simulink model "System_Modell"  (R2018a)
settings: Solver=FixedStepAuto  StartTime=0.0  StopTime=inf  FixedStep=1/f  RelTol=1e-3
values from neighbouring files (symbols this model uses):
  f = 10000    [System_Init.m]
(part 4 of 8)

== matlab function System_Modell/Motor_1/Schnittstelle_0/Recv_2 ==
  data: status input double size=1; clock input double size=1; lenS_1 input; lenS_2 input; lenR input; Rx_2_signal input boolean size=1; Rx_2_data input double size=[1 100]; recv_signal_2 output boolean; recv_package_2 output double size=[1 98]; Send_Buffer_1 data_store_memory; Send_Buffer_2 data_store_memory; T_send_1 data_store_memory; T_recv_1 data_store_memory; De_1 data_store_memory; De_sum_1 data_store_memory; Address data_store_memory; Recv_Buffer data_store_memory; Address_2 data_store_memory; Address_1 data_store_memory; De_sum_2 data_store_memory; Handshake_1 data_store_memory; De_2 data_store_memory; Handshake_2 data_store_memory; T_recv_2 data_store_memory; T_send_2 data_store_memory
% Name: Rx_2

% -------------------------------------------------------------------------------------
% Funktionalitäten:
% Im Init-Prozess
%   1. Handshake durch zu führen
%       103...Handshake ask --> 104 in Send_Buffer_1 additieren
%       104...Handshake answer --> Handshake success
%   2. Delay-Zeit berechnen
%       105...Delay begin --> 106 in Send_Buffer_1 additieren
%       106...Delay end --> Delay_Zeit berechnen
%   3. Sum-Delay-Zeit berechnen
%       107, Receiver = meine Addresse --> Sum_Delay_Zeit berechnen
%       107, Receiver ~= meine Addresse --> Daten in Send_Buffer_2 additieren
% Im normalen Prozess
%   4. Receiver = meine Addresse --> in Recv_Buffer additieren
%   5. Receiver = 255 --> Broadcast --> in Recv_Buffer && Send_Buffer_2 additieren
%   6. Receiver ~= meine Addresse --> in Send_Buffer_2 additieren

% -------------------------------------------------------------------------------------
% Input && Output
% status - status of 'Schnittstelle'
% clock - simulation time
% lenS_2/len_1/lenR - meaningful length of Send_Buffer_2/Send_Buffer_1/Recv_Buffer
% Rx_2_data - from Rx_2 received data
% recv_package_2 - data to send to chart or store in Send_Buffer_2
    % in Init-process, recv_package_2 need to be sent to chart
    % in normal-process, recv_package_2 need to garther all 'to be transmmited' datablock, and store in Send_Buffer_2

function [recv_signal_2, recv_package_2] = Rx_2(status, clock,lenS_1, lenS_2, lenR, Rx_2_signal, Rx_2_data)

global Send_Buffer_2
global Send_Buffer_1
global T_send_2
global T_recv_2
global De_2
%global De_1
global De_sum_2
global Address
global Address_2
%global Address_1
global Recv_Buffer
global Handshake_2

recv_signal_2 = false;
recv_package_2 = zeros(1,98);       % one datablock = [1x7]

lenr = 1;                           % path to write data into recv_package_2

if Rx_2_signal
    a = find(Rx_2_data==102,1);
    len = a(1);
    if ~isempty(len)
        mod_ = mod(len-2,7);
        len_ = ceil((len - 2) / 7);                                 % Round toward positive infinity
    end
    
	if ((mod_ == 0) && (len_ >= 1))                             % package contains at least one datablock
        switch status
            case 1                                              % Handshake
                for i=1:len_
                    switch Rx_2_data(7*i-3)                          % Da.cmd
                        case 103                                % Handshake ask --> send answer
                            check = check_X(104, Address, Send_Buffer_1);
                            if ((Rx_2_data(7*i-5) ~= 0) && (Rx_2_data(7*i-4) == 0) && ~Handshake_2 && ~check)
                                Address_2 = Rx_2_data(7*i-5);
                                Send_Buffer_1(lenS_1:lenS_1+7) = [Address, Address_2, 104, zeros(1,4), 102];
                            end
                        case 104                                % Handshake answer --> Handshake success --> no more send
                            if ((Rx_2_data(7*i-5) ~= 0) && (Rx_2_data(7*i-4) == Address) && ~Handshake_2)
                                Address_2 = Rx_2_data(7*i-5);        % Address of the Host in the Direction_2
                                recv_package_2(lenr:lenr+6) = Rx_2_data(7*i-5:7*i+1);    % [_,_,104,_,_,_,_] = [1x7]
                                lenr = lenr + 7;
                                recv_signal_2 = true;
                            end
                    end
                end

            case 2                                              % Delay_Time_Caculation
                for j=1:len_
                    switch Rx_2_data(7*j-3)                          % Da.cmd
                        case 103                                % Handshake ask --> send answer
                            check = check_X(104, Address, Send_Buffer_1);
                            if ((Rx_2_data(7*j-5) ~= 0) && (Rx_2_data(7*j-4) == 0) && ~Handshake_2 && ~check)
                                Address_2 = Rx_2_data(7*j-5);
                                Send_Buffer_1(lenS_1:lenS_1+7) = [Address, Address_2, 104, zeros(1,4), 102];
                            end
                        case 105                                % Delay ask --> send answer
                            check = check_X(106, Address, Send_Buffer_1);
                            if (isequal(Rx_2_data(7*j-5:7*j-4),[Address_2, Address]) && Handshake_2 && ~check) % check Sender & Receiver
                                Send_Buffer_1(lenS_1:lenS_1+7) = [Address, Address_2, 106, zeros(1,4), 102];
                            end
                        case 106                                % Delay answer --> caculate the time --> no more send
                            if ((isequal(Rx_2_data(7*j-5:7*j-3),[Address_2, Address, 106])) && (De_2 <= 0) && (T_send_2 > 0))
                                T_recv_2 = clock;
                                De_2 = T_recv_2 - T_send_2;
                                T_send_2 = 0;
                                T_recv_2 = 0;
                            end
                    end
                end

            case 3                                              % Sum_Delay_Caculation
                for h=1:len_
                    switch Rx_2_data(7*h-3)
                        case 103                                % Handshake ask --> send answer
                            check = check_X(104, Address, Send_Buffer_1);
                            if ((Rx_2_data(7*h-5) ~= 0) && (Rx_2_data(7*h-4) == 0) && ~Handshake_2 && ~check)
                                Address_2 = Rx_2_data(7*h-5);
                                Send_Buffer_1(lenS_1:lenS_1+7) = [Address, Address_2, 104, zeros(1,4), 102];
                            end
                        case 105                                % Delay ask --> send answer
                            check = check_X(106, Address, Send_Buffer_1);
                            if (isequal(Rx_2_data(7*h-5:7*h-4),[Address_2, Address]) && Handshake_2 && ~check) % check Sender & Receiver
                                Send_Buffer_1(lenS_1:lenS_1+7) = [Address, Address_2, 106, zeros(1,4), 102];
                            end   
                        case 107
                            if (isequal(Rx_2_data(7*h-5:7*h-4),[Address, Address]) && (De_sum_2 <= De_2) && (T_send_2 > 0))                   % Sum_Delay --> caculate the time --> no more send
                                T_recv_2 = clock;
                                De_sum_2 = T_recv_2 - T_send_2;
                                T_send_2 = 0;
                                T_recv_2 = 0;
                            elseif ((isequal(Rx_2_data(7*h-5),Rx_2_data(7*h-4))) && (Rx_2_data(7*h-5) ~= Address))
                                check = check_Y(Rx_2_data(7*h-5:7*h), recv_package_2) || check_Y(Rx_2_data(7*h-5:7*h), Send_Buffer_2);
                                if ~check
                                    recv_package_2(lenr:lenr+6) = Rx_2_data(7*h-5:7*h+1)';
                                    lenr = lenr + 7;
                                end
                            end
                    end
                end
                Send_Buffer_2(lenS_2:lenS_2+lenr-1) = [recv_package_2(1:lenr-1),102];           % 前提：lenS更新速度比当前更新快

            case 4                                               % normal communication between all Hosts
                for k=1:len_
                    switch Rx_2_data(7*k-3)
                        case 103                                % Handshake ask --> send answer
                            check = check_X(104, Address, Send_Buffer_1);
                            if ((Rx_2_data(7*k-5) ~= 0) && (Rx_2_data(7*k-4) == 0) && ~Handshake_2 && ~check)
                                Address_2 = Rx_2_data(7*k-5);
                                Send_Buffer_1(lenS_1:lenS_1+7) = [Address, Address_2, 104, zeros(1,4), 102];
                            end
                        case 105                                % Delay ask --> send answer
                            check = check_X(106, Address, Send_Buffer_1);
                            if (isequal(Rx_2_data(7*k-5:7*k-4),[Address_2, Address]) && Handshake_2 && ~check) % check Sender & Receiver
                                Send_Buffer_1(lenS_1:lenS_1+7) = [Address, 0, 106, zeros(1,4), 102];
                            end
                        case 107
                            if ((isequal(Rx_2_data(7*k-5),Rx_2_data(7*k-4))) && (Rx_2_data(7*k-5) ~= Address))
                                check = check_Y(Rx_2_data(7*k-5:7*k), recv_package_2) || check_Y(Rx_2_data(7*k-5:7*k), Send_Buffer_2);
                                if ~check
                                    recv_package_2(lenr:lenr+6) = Rx_2_data(7*k-5:7*k+1)';
                                    lenr = lenr + 7;
                                end
                            end
                        otherwise
                            if ((Rx_2_data(7*k-5) ~= Address) && (Rx_2_data(7*k-4) == Address))   % Datablock sent to me --> store in Recv_Buffer
                                check = check_Y(Rx_2_data(7*k-5:7*k), Recv_Buffer');
                                if ~check
                                    Recv_Buffer(lenR+1,:) = Rx_2_data(7*k-5:7*k+1);
                                end
                            elseif ((Rx_2_data(7*k-5) ~=Address) && (Rx_2_data(7*k-4) == 255))    % Datablock is as a Broadcast --> store in Recv_Buffer && Send_Buffer_2
                                check = check_Y(Rx_2_data(7*k-5:7*k), Recv_Buffer');
                                if ~check
                                    Recv_Buffer(lenR+1,:) = Rx_2_data(7*k-5:7*k+1);
                                end
                                check = check_Y(Rx_2_data(7*k-5:7*k), recv_package_2) || check_Y(Rx_2_data(7*k-5:7*k), Send_Buffer_2);
                                if ~check
                                    recv_package_2(lenr:lenr+6) = Rx_2_data(7*k-5:7*k+1)';
                                    lenr = lenr + 7;
                                end
                            elseif ((Rx_2_data(7*k-4) ~= Address) && (Rx_2_data(7*k-4) ~= 255))   % Datablock not sent to me --> to transmmit --> store in Send_Buffer_2
                                check = check_Y(Rx_2_data(7*k-5:7*k), recv_package_2) || check_Y(Rx_2_data(7*k-5:7*k), Send_Buffer_2);
                                if ~check
                                    recv_package_2(lenr:lenr+6) = Rx_2_data(7*k-5:7*k+1)';
                                    lenr = lenr + 7;
                                end
                            end
                    end
                end
                Send_Buffer_2(lenS_2:lenS_2+lenr-1) = [recv_package_2(1:lenr-1),102];
        end
	elseif mod_ ~= 0
        fprintf("Eroor: Package length not avalueable!");
	end
end

end

% check_X: to check if Data contains a Datablock with CMD and adr
function y = check_X(CMD, adr, Data)          % y: boolean; x: double, [1x100];

x = find(Data==CMD);
y = (~isempty(x));

if y
    y = y && (Data(1,x(1)-2) == adr);
end

end

% check_Y: to check if Data contains data
function y = check_Y(data, Data)          % y: boolean; data: double, [1x6];

x = find(Data==data(3));
y = (~isempty(x));
if y
    for i=1:length(x)
        if(isequal(Data(x(i)-2:x(i)+3),data))
            y = true;
            break
        else
            y = false;
        end
    end
end

end

== matlab function System_Modell/Motor_1/Schnittstelle_0/Send_Telegram/Send_Telegram_1 ==
  data: status input double size=1; clock input double; lenS_1 input; impulse input boolean size=1; Tx_1_signal output boolean size=1; Tx_1_data output double size=[1,100]; send_1_old input boolean size=1; T_send_1 data_store_memory; T_send_2 data_store_memory; Send_Buffer_1 data_store_memory; Send_Buffer_2 data_store_memory; De_1 data_store_memory; De_2 data_store_memory; De_sum_1 data_store_memory; De_sum_2 data_store_memory; Address data_store_memory
% Name: send_telegram
% Funktionalität:
% Datenpacket in Send_Buffer_1 und Send_Buffer2 zyklisch transferieren.
% Die Zykluszeit lautet 10ms

function [Tx_1_signal, Tx_1_data] = send_telegram_1(status, clock, lenS_1, impulse, send_1_old)

global Send_Buffer_1
global De_1
global De_sum_1
global T_send_1
global Address

timer_1 = 0;

if send_1_old
    % The Send_Signal lasts for only one period. Then it need to be shut down.
    Tx_1_signal = false;
    Tx_1_data = [101,102,zeros(1,98)];
else
    % No Error + send-signal already shut down + Impulse-Signal --> OK! Let's send the telegram!
    h1 = ceil((lenS_1 - 2) / 7);
    if ((status > 0) && (~send_1_old) && impulse && (h1 > 0))
        % Before send, we need check if we need to do something else. For example: 'start the Timer' or 'caculate a new De in each datablock'
        switch status
            case 2                                              % Delay time caculation
                if ~isempty(find(Send_Buffer_1==105,1))                     % check if there is a 105-cmd in Send_Buffer,if so, timer need to be started
                    timer_1 = 1;
                end

            case 3                                              % Sum_Delay caculation
                for i1=1:h1
                    if isequal([Send_Buffer_1(7*i1-5:7*i1-3),De_sum_1],[Address,Address,107,0])     % check if there is a 107-cmd in Send_Buffer
                        timer_1 = 1;
                        break
                    end
                end

            case 4
                for i1=1:h1                                                    % recaculate the Delay time for each datablock
                    Send_Buffer_1(7*i1+1) = Send_Buffer_1(7*i1+1) + De_1;
                end
        end
        
        % Now we can send the telegram!!
        Tx_1_data = Send_Buffer_1;                                  % send data
        Tx_1_signal = true;
        
        % remember the send-time if necessary
        if timer_1 == 1
            T_send_1 = clock;
        end
        
        % clear the data in Send_Buffer after sending
        Send_Buffer_1 = [101,102,zeros(1,98)];

    else
        Tx_1_signal = false;
        Tx_1_data = [101,102,zeros(1,98)];
    end
end

end

== matlab function System_Modell/Motor_1/Schnittstelle_0/Send_to_Host ==
  data: signal output boolean size=1; package output double; Recv_Buffer data_store_memory; Filter data_store_memory; lenR input; lenF input; signal_old input
% Name: Send_to_Host
% Funktionalitäten:
% 1. Erste Zeile der Nachricht von Recv_Buffer in Filter prüfen
% 2. nicht wiederholte Nachricht an Host senden
% 3. wiederholte Nachricht in Filter löschen
% 4. gesendete Nachricht in Filter kopieren
% 5. folgende Nachrichten eine Zeile nach oben verschoben


function [signal, package] = send_to_Host(lenR, lenF, signal_old)

global Recv_Buffer          % Package-List, which will be sent to the Host
global Filter               % Package-List, which has been sent to the Host

package = zeros(1,7);
check = 0;

if signal_old               % signal can only last for one periode
    signal = false;
    package = zeros(1,7);

else                        % signal inactiv --> now we can send new data to host.
    if (lenR >= 1)
        if lenF >= 1        % check in Filter
            for i=1:lenF        % check if the same message sent before
                if isequal(Recv_Buffer(1,:),Filter(i,:))
                    check = i;
                    break
                else
                    check = 0;
                end
            end
        end
        
        if check ~= 0       % same message in Filter found --> delete the message in Recv_Buffer and Filter
            signal = false;
            package = zeros(1,7);
            Filter(check:lenF-1,:) = Filter(check+1:lenF,:);
            Filter(lenF,:) = zeros(1,7);
            Recv_Buffer(1:lenR-1,:) = Recv_Buffer(2:lenR,:);
            Recv_Buffer(lenR,:) = zeros(1,7);
        else                % same message in Filter not found --> send to Host --> copy the message in Filter delete it in Recv_Buffer
            package = Recv_Buffer(1,:);
            signal = true;
            Filter(lenF+1,:) = Recv_Buffer(1,:);    % copy
            Recv_Buffer(1:lenR-1,:) = Recv_Buffer(2:lenR,:);    % delete
            Recv_Buffer(lenR,:) = zeros(1,7);
        end
    else
        signal = false;
        package = zeros(1,7);
    end
end


end

== stateflow chart System_Modell/Motor_1/Schnittstelle_0/Status ==
  state Init_0
    entry:	status=0;
    Handshake_1=false;
    Handshake_2=false;
    De_1 = 0;
    De_2 = 0;
    De_sum_1 = 0;
    De_sum_2 = 0;
    Filter(1,:) = zeros(1,7);
  state Error
    entry: status=-2;
  note: 未初始化全局变量
  state Init_1_Handshake
    entry: status=1;
  state Init_2_Delay_Time
    entry:	status=2;
  state Init_3_Sum_Delay_Time
    entry:	status=3;
  state Run
    entry: status=4;
  (default) -> Init_0
  Error -> Init_0 : [~Error_Signal]
  Init_0 -> Init_1_Handshake
  Init_1_Handshake -> Error [order 3] : [Error_Signal]
  Init_1_Handshake -> (junction 75) [order 1] : [recv_signal_1]
  (junction 75) -> Init_1_Handshake : [recv_data_1(1,3)==104]{Handshake_1 = true;}
  Init_1_Handshake -> (junction 77) [order 2] : [recv_signal_2]
  (junction 77) -> Init_1_Handshake : [recv_data_2(1,3)==104]{Handshake_2 = true;}
  Init_1_Handshake -> Init_2_Delay_Time [order 4] : [Handshake_1 && Handshake_2 && Address_1 > 0 && Address_2 > 0]
  Init_2_Delay_Time -> Error [order 2] : [Error_Signal]
  Init_2_Delay_Time -> Init_3_Sum_Delay_Time [order 1] : [De_1>0 && De_2>0]
  Init_3_Sum_Delay_Time -> Error [order 2] : [Error_Signal]
  Init_3_Sum_Delay_Time -> Run [order 1] : [De_sum_1 > De_1 && De_sum_2 > De_2]
  Run -> Error : [Error_Signal]
  data: status output double size=1; Error_Signal input boolean size=1; recv_signal_1 input boolean size=1; recv_data_1 input double; Handshake_1 data_store_memory size=1; Handshake_2 data_store_memory size=1; De_1 data_store_memory; De_2 data_store_memory; De_sum_1 data_store_memory; De_sum_2 data_store_memory; recv_signal_2 input boolean; recv_data_2 input double; Address_1 data_store_memory; Address_2 data_store_memory; Filter data_store_memory

== stateflow chart System_Modell/Motor_2/CommSM_1/Status_Control ==
  state Init
    entry: 	status=1;
    send_AT_package=[Adresse, zeros(1,6)];
    send_signal=false;
    send_MotionSM=[0,0];
  state Aus
    entry: status=0;
  state Ein
    state State_Control [parallel]
      settings: executionOrder=1
      note: % Protokoll
          | % SummenTelegramm = [HDR, SDT, END]
          | %HDR: header, SDT: Summen-Daten-Telegramm, END: Ender
          |
          | % SDT = [SDT_7, SDT_1, SDT_2, SDT_3]
          | % SDT_i = [Da_i, De_i]
          | %Da: Data, De: Delay
          | %i...{1,2,3,7} %7...GSM, 1-3...CommSM1-3
          |
          | % Da_i = [sender, receiver, cmd, N, ZP, ZP_status]
          | %sender,receiver...{1,2,3,7,255} %255...Broadcast
          | %cmd: 1...addP, 2...getP, 3...setS, 4...getS
          | %ZP_status: 0...none, 1...wait, 2...active, 3...done, 4...error
          |
          | % Da_i = [sender, receiver, cmd, N, s , s _status]
          | %cmd: 5 ...negO
          | % s _status: 0...none, 1...negotiation, 2...excute, 3...done
      note: 问题
          | 如何检测下一个新的ZP
      state send_AT_2_GSM
        entry:	status=16;
        permission=true;
        send_AT_package=[Adresse, 7, 113, ZPT(N,1:3), 0];
        %AT=[CommSM, GSM, setS, n, ZP, done];
        send_signal=true;
      state Free
        entry:	status=2;
      state Arrival
        entry:	status=15;
        ZPT(N,3)=3;
      state check_ZPT
        entry:	status=3;
        ZPT(N,3)=2;	      % status='active'
      state wait_arrival
        entry: status=14
      state send_Status_activ
        entry:	status=4;
        permission = true;
        send_AT_package = [Adresse, 7, 113, ZPT(N,1:3), 0];
        % AT=[CommSM, GSM, setS, n, ZP, activ];
        send_signal = true;
      state check_ZP
        entry: 	status=5;
        s=checkZP(ZZP_old, Adresse, N);
        % s-range: [0, 100], ZZP_old: ZZP for last loop
      state MotionSM
        entry:	status=13;
        send_MotionSM=[3, ZZPT(Adresse,2)];	%excute ZZP
        a = ZPT(N,2); b = ZZPT(Adresse,2);
      state send_nego_1
        entry: 	status=6;
        permission = true;
        send_AT_package=[Adresse, 255, 115, ZPT(N,1), s, 1, 0];
        % AT=[CommSM, Broadcast, negO, n, s, nego];
        send_signal=true;
      state Nego_wait
        entry: 	status=7;
      state send_excu
        entry:	status=12;
        permission = true;
        send_AT_package = [Adresse, 255, 115, ZPT(N,1), ZZPT(Adresse, 4), 2, 0];
        %AT=[CommSM, Broadcast, negO, n, s, excu];
        send_signal = true;
      state Wait_excution
        entry:	status=11;
        send_MotionSM=[1, ZZPT(Adresse,2)]; %set ZZP
      state s_Compair
        entry: 	status=8;
        s_new=s_compair(Adresse);
      state status_excution
        entry: 	status=10;
        ZZPT(Adresse,4)=2; %excu
      state ZZP_new
        entry:	status=9;
        ZZPT(Adresse,3)=s_new;
        ZZPT(Adresse,2)=AP+(ZPT(N,2)-AP)*(s_new/100);
      (default) -> Free
      send_AT_2_GSM -> Free : [send_done]{send_signal=false; permission = false;}
      Free -> check_ZPT : % status ='wait' && MotionSM kein Fehler
          | [N>0 && ZPT(N,3)==1 && status_MotionSM>=1]{send_signal = false;}
      (junction 77) -> send_AT_2_GSM : [~permission]
      Arrival -> (junction 77)
      (junction 121) -> (junction 77)
      wait_arrival -> Arrival : % ZP == ZZP -> wait until ZP == AP
          | [isequal([ZPT(N,2), status_MotionSM],[AP, 2])]
          | {ZZPT=zeros(3,4);}
      check_ZPT -> send_Status_activ : [ZPT(N,3)==2 && ~permission]
      MotionSM -> wait_arrival [order 2] : % ZP == ZZP -> ZP will be arrived & no next ZP -> end
          | [status_MotionSM==3 && a==b && isempty(find(ZPT(:,3)==1,1))]
          | {send_MotionSM=zeros(1,2)}
      (junction 116) -> (junction 99)
      (junction 148) -> (junction 116)
      send_Status_activ -> (junction 99) : [send_done]{send_signal = false; permission = false;}
      (junction 99) -> check_ZP
      MotionSM -> (junction 116) [order 1] : % ZP~=ZZP -> ZP will not be arrived -> negotiate again
          | [status_MotionSM==3 && a~=b]
          | {ZZP_old = ZZPT(Adresse,2); ZZPT = zeros(3,4);}
      MotionSM -> (junction 148) [order 3] : [false]
          | % ZP = ZZP -> ZP will be arrived -> new ZP wait to negotiate -> loop
          | %[status_MotionSM==3 && a==b && ~isempty(find(ZPT(:,3)==1,1))]
          | %{ZZP_old = ZZPT(Adresse,2); ZZPT = zeros(3,4)}
      check_ZP -> send_nego_1 : [~permission]
      (junction 146) -> MotionSM : % Motor stoped
          | [status_MotionSM==2]
      (junction 216) -> (junction 146) : % all axis excuteable && received ZZP from MotionSM
          | [isequal(ZZPT(1:3,4),[2;2;2]) && isequal(data_from_MotionSM(1:2),[2,ZZPT(Adresse,2)])]
          | {ZZP_old=0;}
      send_nego_1 -> Nego_wait : [send_done]{s=0; send_signal=false; permission = false;}
      send_excu -> (junction 216) : [send_done]{send_signal=false; permission = false;}
      Nego_wait -> (junction 121) [order 1] : % ZP = AP, ZP schon erreicht
          | [ZPT(N,3)==3]
      Nego_wait -> (junction 134) [order 2] : % ZP~=AP, ZP "activ"
          | [ZPT(N,3)==2]
      Wait_excution -> send_excu : [~permission]
      (junction 134) -> s_Compair : % ob ZZPT komplett erfüllt
          | [isequal(ZZPT(1:3,1),[1,1,1]')]
      status_excution -> Wait_excution : [status_MotionSM>=2]  % 2 or 3
      s_Compair -> (junction 79)
      (junction 66) -> status_excution : {s_new=0;}
      (junction 79) -> (junction 66) [order 2] : [s_new>=ZZPT(Adresse,3)]
      (junction 79) -> ZZP_new [order 1] : [s_new<ZZPT(Adresse,3)]
      ZZP_new -> (junction 66)
    state Send [parallel]
      settings: executionOrder=2
      state wait
      state send
        entry: permission = true;
        send_AT_package = [Adresse, 7, 2, ZPT(n-1,1:3),0];
        send_signal = true;
      (default) -> wait
      wait -> (junction 181) : % Requirement to respond GSM
          | [respond]
      send -> wait : % send done
          | [send_done]{respond = false;send_signal = false; permission = false;}
      (junction 181) -> send : % permission to use send_port
          | [~permission]
  state Error
    entry: status=-1;
  (default) -> Aus
  Aus -> Init : [EinAus && ~NotAus && ~ErrorSignal]
  Init -> Aus [order 2] : [~EinAus]
  Init -> Error [order 3] : [NotAus]
  Error -> Aus [order 1] : [~EinAus]
  Ein -> Aus [order 1] : [~EinAus]
  Error -> Init [order 2] : [Richten && ~NotAus && ~ErrorSignal]
  Init -> Ein [order 1] : [status_Schnittstelle==4]{send_signal=false;}
  Ein -> Error [order 2] : [NotAus]
  data: zzp_old function_input double size=1; S function_output; adress function_input double size=1; N_ function_input; S_new function_output double size=1; nr function_input double size=1; Adresse input double size=1; status_Schnittstelle input double size=1; n input; N input; NotAus input boolean size=1; EinAus input boolean size=1; Richten input boolean size=1; ErrorSignal input boolean size=1; send_done input; status output double size=1; send_signal output boolean size=1 =false; send_AT_package output double size=[1,7] =zeros(1,7); status_MotionSM input double size=1; data_from_MotionSM input double size=[1,2]; ZPT data_store_memory; ZZPT data_store_memory; AP data_store_memory; s local double size=1 =0; s_new local double size=1 =0; send_MotionSM output double size=[1,2] =zeros(1,2); ZZP_old local double size=1 =0; permission local boolean size=1 =false; respond data_store_memory; a local; b local
  function S = checkZP(zzp_old, adress, N_):
    | %ZPT = [10x3], [ZP_Nr., ZP, status]
    | %status: {0...none, 1...wait, 2...active, 3...done, 4...error}
    | 
    | %ZZPT(CommSM_i,:) = [ZP-Nr., ZZP, s%, status]
    | %status: {0...none, 1...negotiation, 2...excution, 3...done}
    | 
    | function S = checkZP(zzp_old, adress, N_)
    | %1. prüfen, ob ZP unter begrenzte Bedienung erreichbar ist
    |         %Ja     --> ZZP = ZP
    |         %Nein   --> neuen ZZP erzeugen
    | %2. neu ausgerechnete ZZP in der ZZP Tabelle einschreiben
    |  
    | global AP
    | global ZPT
    | global ZZPT
    | 
    | a_max = 1000;   % mm/s^2
    | v_max = 1000;   % mm/s
    | d_T = 10;    % s
    | 
    | s_max = a_max*d_T*d_T/4;
    | if zzp_old <= 0             %last ZZP to arrive. After the Motor is started, ZZP_old = ZZP, ZZPT = zeros(3,4);
    |     s0 = ZPT(N_,2) - AP;     %ZP - AP
    | else
    |     s0 = ZPT(N_,2) - zzp_old;    %excist last ZZP
    | end
    | 
    | if abs(s0) <= s_max
    |     S = 100;                    % 100% erreichbar
    | elseif abs(s0) > 0 && abs(s0) < 100
    |     S = abs(100*s_max/s0);      % s% s: [0, 100]
    |     S = fix(1000*S)/1000;       % Genauigkeit = 10000*0.001%=0.1 mm
    | else
    |     S = 0;                      % ZP = AP, Achse keine Bewegung
    | end
    | 
    | %ZZP-Tabelle erfüllen
    | if zzp_old <= 0
    |     ZZP_new = AP + s0*S/100;        %neue ZZP in der ZZP-Tabelle einschreiben
    | else
    |     ZZP_new = zzp_old+s0*S/100;
    | end
    | 
    | if S == 0
    |     ZPT(N_,3) = 3;
    | else
    |     ZZPT(adress,:) = [ZPT(N_,1), ZZP_new, S, 1];
    | end
    | 
    | end
  function S_new = s_compair(nr):
    | function S_new = s_compair(nr)
    | 
    | global ZZPT
    | 
    | s_ = ZZPT(:,3);
    | 
    | S_new = s_(nr);          % CommSM_me
    | 
    | for i = 1:3                         % s==0 --> s=100
    |     if i ~= nr && s_(i)== 0
    |         s_(i) = 100;
    |     end
    | end
    | 
    | s_min = min(s_);
    | if S_new > s_min
    |     S_new = s_min;
    | end
    | 
    | end

== stateflow chart System_Modell/Motor_2/MotionSM_1/Chart ==
  state Off
    entry: status=0;
  state Init
    entry: status=1; parameter=Par_1(delta_T);
  state On
    state Stop
      entry: status=2;
    state Run
      entry: status=3;
    (default) -> Stop
    Stop -> Run : [excute_signal==1 && ZZP~=AP && Motor_status == 0]
        | {parameter=Par(delta_T);}
    Run -> Stop : [ZZP==AP && ~Motor_status]
  state Error
    entry: status=-1;
  (default) -> Off
  Init -> Off [order 1] : [~EinAus]
  Off -> Init [order 2] : [EinAus && ~ NotAus]{parameter=[delta_T,0,0,0]';}
  Init -> Error [order 2] : [Motor_status==-1 || NotAus || ErrorSignal]
  Off -> Error [order 1] : [EinAus && (ErrorSignal || NotAus)]
  Error -> Off [order 1] : [~EinAus]
  On -> Off [order 1] : [~EinAus]
  Error -> Init [order 2] : [Richten]{parameter=[delta_T,0,0,0]';}
  Init -> On [order 3] : [AP==0]{parameter=[delta_T,0,0,0]';}
  On -> Error [order 2] : [Motor_status==-1 || NotAus || ErrorSignal]
  data: par function_output double size=4; delta_t function_input double size=1; par function_output double size=4; delta_t function_input double size=1; NotAus input boolean size=1; EinAus input boolean size=1; Richten input boolean size=1; ErrorSignal input boolean size=1; excute_signal input boolean size=1; Motor_status input boolean size=1; status output double size=1 =0; ZZP data_store_memory; ZZP_wait data_store_memory; parameter output double size=4; AP data_store_memory size=1; delta_T input double size=1
  function par = Par_1(delta_t):
    | function par = Par_1(delta_t)
    | 
    | global ZZP
    | global ZZP_wait
    | global AP
    | 
    | % delta_T = 10 s
    | ZZP = 0;
    | ZZP_wait = 0;
    | s0 = ZZP - AP;
    | a_max = 100;        % 1 m/s^2
    | v_max = 1;
    | %v_max = 0.5 * a_max * (delta_t - sqrt(delta_t*delta_t - 4*abs(s0)/a_max));   	% mm/s
    | 
    | par = [delta_t, a_max, v_max, s0]';
    | end
  function par = Par(delta_t):
    | function par = Par(delta_t)
    | 
    | global ZZP
    | global AP
    | 
    | s0 = ZZP - AP;
    | a_max = 1000;       % 1 m/s^2
    | v_max = 0.5 * a_max * (delta_t - sqrt(delta_t*delta_t - 4*abs(s0)/a_max));  % mm/s
    | 
    | par = [delta_t, a_max, v_max, s0]';
    | end

== stateflow chart System_Modell/ZP_Mananger/GSM /State Machine ==
  settings: executeAtInitialization=1
  state Off
    entry: status = 0;
  state Error
    entry: status = -2;
  state Init
    entry: status = 1;
  state Run
    state Send_ZP
      entry:	status = 3;
      Data_Package = SkillRequest_package;
      send_signal = true;
    state Stand_By
      entry: status = 2;
    state ZP_Status_Update
      entry:	status = 4;
      Update_signal = received_signal;
    note: ZP_Status_Update = [address, command, n, Ax, status]
    note: received_package = [address, command, n, Ax, status]
    (default) -> Stand_By
    Stand_By -> Send_ZP [order 1] : [SkillRequest_signal]
    Send_ZP -> Stand_By : [~SkillRequest_signal]{send_signal=false;}
    ZP_Status_Update -> Stand_By : [update_done && ~received_signal]{Update_signal=false;}
    Stand_By -> ZP_Status_Update [order 2] : [received_signal && ~update_done]
  (default) -> Off
  Error -> Off [order 1] : [~EinAus]
  Off -> Error [order 2] : [EinAus && NotAus]
  Init -> Off [order 3] : [~EinAus]
  Off -> Init [order 1] : [EinAus && ~NotAus]
  Error -> Init [order 2] : [~GSM_Error && Richten] {GSM_ErrorCode=0;}
  Init -> Error [order 1] : [GSM_Error || NotAus]{GSM_ErrorCode=status}
  Run -> Init [order 2] : [Schnittstelle_status~=4 && ~GSM_Error]
  Init -> Run [order 2] : [Schnittstelle_status==4]
  Run -> Error [order 1] : [GSM_Error || NotAus]{GSM_ErrorCode=status}
  data: NotAus input boolean; EinAus input boolean; Richten input boolean; GSM_Error input boolean; SkillRequest_signal input boolean; SkillRequest_package input double; Schnittstelle_status input double; status output double; send_signal output boolean; received_signal input boolean; update_done input boolean; Data_Package output double; GSM_ErrorCode output double; Update_signal output boolean size=1

== matlab function System_Modell/ZP_Mananger/GSM /ZP-Tabelle bearbeiten/MATLAB Function ==
  data: address input; update_signal input boolean; update_data input double size=7; ZP_update_done output boolean; ZP_Tabelle data_store_memory
%ZP_to_update = [address, command, n, Ax, status]

function ZP_update_done  = Status_Update(address, update_signal, update_data)

global ZP_Tabelle

if (update_signal && (update_data(2) == address))
    
    Y = 2 * update_data(1) + 1;             % Matrix-Index berechnen
    n = update_data(4);                     % ZP_n
    position = update_data(5);
    status = update_data(6);
    
    X = find(ZP_Tabelle(:,1)==n,1);	%ZP_N bestimmen
    if (~isempty(X) && isequal(ZP_Tabelle(X(1),Y-1),position))
        if ((status == -2) || ZP_Tabelle(X(1),Y) <= status)
            ZP_Tabelle(X(1),Y) = status;
        end
    end
    ZP_update_done = true;
    
else
    ZP_update_done = false;
    
end

end

== matlab function System_Modell/ZP_Mananger/GSM /ZP-Tabelle bearbeiten/add_new_ZP/add_new_ZP ==
  data: adr input; SkillRequest input; SkillRequest_last input; n input; send_SkillRequest output double; SkillRequest_remember output; n_remember output; ZP_Tabelle data_store_memory
% neu SkillRequest in ZP-Tabelle eintragen
% Sendpackage erstellen

function [send_SkillRequest, SkillRequest_remember, n_remember] = add_new_ZP(adr, SkillRequest, SkillRequest_last, n)

global ZP_Tabelle

if ~isequal(SkillRequest,SkillRequest_last)   % same position filtern
    X = min(find(ZP_Tabelle(:,1)==0,1));      % find the first free line
    if ~isempty(X)
        ZP_Tabelle(X,:) = [n, SkillRequest(1), 1, SkillRequest(2), 1, SkillRequest(3), 1];  % add new ZP in the ZP-Tabelle
        send_SkillRequest = [adr,1,111,n,SkillRequest(1),1,0, adr,2,111,n,SkillRequest(2),1,0, adr,3,111,n,SkillRequest(3),1,0]; % create new ZP package
        n_remember = n;
    end
else
    send_SkillRequest = zeros(1,21);
    n_remember = n-1;
end

SkillRequest_remember = SkillRequest;
end

== matlab function System_Modell/ZP_Mananger/Schnittstelle_1/Add_to_Send_Buffer ==
  data: Send_Buffer_1 data_store_memory; Send_Buffer_2 data_store_memory; Address data_store_memory; status input; lenS_1 input; lenS_2 input; to_send_signal input; to_send_package input; Address_1 data_store_memory; Address_2 data_store_memory; Handshake_1 data_store_memory; Handshake_2 data_store_memory; Filter data_store_memory; De_1 data_store_memory; De_2 data_store_memory; De_sum_1 data_store_memory; De_sum_2 data_store_memory
% Name: add_to_Send_Buffer
% Funktionalitäten
% Handshake-Message einfügen, wenn Status==1
% Delay-caculation-Message einfügen, wenn Status==2
% Sum-Delay-caculation-Message einfügen, wemm Status==3
% Nachrichten, die der Host senden möchte, einfügen, wenn Status==4

function add_to_Send_Buffer(status, lenS_1, lenS_2, to_send_signal, to_send_package)

global Send_Buffer_1
global Send_Buffer_2
global Address
global Address_1
global Address_2
global Handshake_1
global Handshake_2
global Filter
global De_1
global De_2
global De_sum_1
global De_sum_2

switch status
    case -2                         % Error Signal einrichten
        Filter(1,7) = 1;
    case 1                          % Handshake
        if((Filter(1,1) == 0) && ~Handshake_1)              % 103 not sent yet || Handshake_1 not finish yet
            check_1 = check_X(103, Address, Send_Buffer_1);          % check if there is a 103-Message in Send_Buffer_1
            if ~check_1
                Send_Buffer_1(lenS_1:lenS_1+7) = [Address, 0, 103, zeros(1,4), 102];
                Filter(1,1) = 1;                            % to remember, if 103 ist sent
            end
        end
        if((Filter(1,2) == 0) && ~Handshake_2)
            check_2 = check_X(103, Address, Send_Buffer_2);
            if ~check_2
                Send_Buffer_2(lenS_2:lenS_2+7) = [Address, 0, 103, zeros(1,4), 102];
                Filter(1,2) = 1;
            end
        end

        
    case 2                          % Delay time caculation
        if((Filter(1,3) == 0 ) && (De_1 <= 0))              % 105 not sent || De_1 not caculated yet
            check_1 = check_X(105, Address, Send_Buffer_1);
            if ~check_1
                Send_Buffer_1(lenS_1:lenS_1+7) = [Address, Address_2, 105, zeros(1,4), 102];
                Filter(1,3) = 1;
            end
        end
        if((Filter(1,4) == 0 ) && (De_2 <= 0))
            check_2 = check_X(105, Address, Send_Buffer_2);
            if ~check_2
                Send_Buffer_2(lenS_2:lenS_2+7) = [Address, Address_1, 105, zeros(1,4), 102];
                Filter(1,4) = 1;
            end
        end
        
    case 3                          % Sum_Delay caculation
        if((Filter(1,5) == 0 ) && (De_sum_1 <= 0))          % 107 not sent || De_sum_1 not caculated yet
            check_1 = check_X(107, Address, Send_Buffer_1);
            if ~check_1
                Send_Buffer_1(lenS_1:lenS_1+7) = [Address, Address, 107, zeros(1,4), 102];
                Filter(1,5) = 1;
            end
        end
        if((Filter(1,6) == 0 ) && (De_sum_2 <= 0))
            check_2 = check_X(107, Address, Send_Buffer_2);
            if ~check_2
                Send_Buffer_2(lenS_2:lenS_2+7) = [Address, Address, 107, zeros(1,4), 102];
                Filter(1,6) = 1;
            end
        end
        
    case 4                          % normal communication
        if to_send_signal
            check_1 = check_Y(to_send_package, Send_Buffer_1);
            check_2 = check_Y(to_send_package, Send_Buffer_2);
            if ~check_1
                Send_Buffer_1(lenS_1:lenS_1+21) = [to_send_package, 102];       % Attention!!!! 21 is the lenth of cariable 'wait_to_send'
            end
            if ~check_2
                Send_Buffer_2(lenS_2:lenS_2+21) = [to_send_package, 102];
            end
        end
end

end

function y = check_X(CMD, adr, Data)          % y: boolean; x: double, [1x100];

x = find(Data==CMD);
y = ~isempty(x);
if y
    y = y && (Data(1,x(1)-2) == adr);
end

end

function y = check_Y(data, Data)          % y: boolean; data: double, [1x6];

x = find(Data==data(3));        % CMD
y = ~isempty(x);
if y
    for i=1:length(x)
        if(isequal(Data(x(i)-2:x(i)+3),data(1:6)))
            y = true;
            break
        else
            y = false;
        end
    end
end

end

== matlab function System_Modell/ZP_Mananger/Schnittstelle_1/Global_Var_Length ==
  data: len_Send_Buffer_1 output double size=1; len_Send_Buffer_2 output double size=1; len_Recv_Buffer output double size=1; len_Filter output double size=1; Send_Buffer_1 data_store_memory; Send_Buffer_2 data_store_memory; Recv_Buffer data_store_memory; Filter data_store_memory
% genutzte Länge der globale Variablen berechnen

function [len_Send_Buffer_1, len_Send_Buffer_2, len_Recv_Buffer, len_Filter] = Length
global Send_Buffer_1
global Send_Buffer_2
global Recv_Buffer
global Filter

a1 = find(Send_Buffer_1==102,1);
len_Send_Buffer_1 = a1(1);
a2 = find(Send_Buffer_2==102,1);
len_Send_Buffer_2 = a2(1);

len_Recv_Buffer = min(find(Recv_Buffer==0,150))-1;
len_Filter = min(find(Filter(2:20)==0,150));

end
